simulink model "TwoButtonReaction"  (R2023b)
settings: Solver=FixedStepAuto  StartTime=0.0  StopTime=Inf  FixedStep=0.001  RelTol=1e-3  EnableMultiTasking=on
libraries: arduinolib x5
settings Model: ExtModeTrigDuration=2  Creator=vboutrou  LastModifiedBy=vboutrou
settings DataIOCC: DSMLogging=off  SaveTime=off  ReturnWorkspaceOutputs=off
settings OptimizationCC: EnhancedBackFolding=on  PassReuseOutputArgsAs=Individual arguments  ZeroExternalMemoryAtStartup=off  ZeroInternalMemoryAtStartup=off  MaxStackSize=64  OptimizeBlockOrder=speed  DifferentSizesBufferReuse=on  OptimizationCustomize=off  EfficientTunableParamExpr=on
settings DebuggingCC: ParameterTunabilityLossMsg=error
settings HardwareCC: ProdBitPerInt=16  ProdBitPerPointer=16  ProdBitPerSizeT=16  ProdBitPerPtrDiffT=16  ProdLargestAtomicFloat=None  ProdWordSize=8  ProdHWDeviceType=Atmel->AVR
settings SFSimCC: MATLABDynamicMemAlloc=off
settings RTWCC: Description=Embedded Coder  SystemTargetFile=ert.tlc  HardwareBoard=Arduino Uno  TemplateMakefile=ert_default_tmf  Toolchain=Arduino AVR  BuildConfiguration=Faster Runs
settings CodeAppCC: ForceParamTrailComments=on  IgnoreCustomStorageClasses=off  MaxIdLength=95  OperatorAnnotations=on  SimulinkDataObjDesc=on  SFDataObjDesc=on  InsertBlockDesc=on
settings ERTTargetCC: SupportContinuousTime=on  SupportVariableSizeSignals=on  ExtModeTransport=3  ExtModeStaticAlloc=on  ExtModeAutomaticAllocSize=off  ExtModeStaticAllocSize=250  ExtModeMexFile=ext_xcp  ExtModeIntrfLevel=Level2 - Open

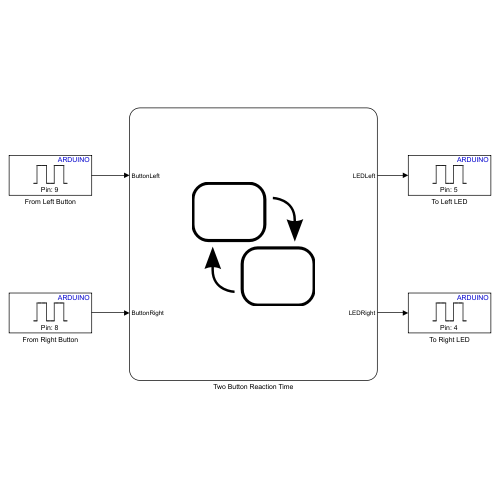
[thumbnail: Simulink's stored preview of the top-level diagram]
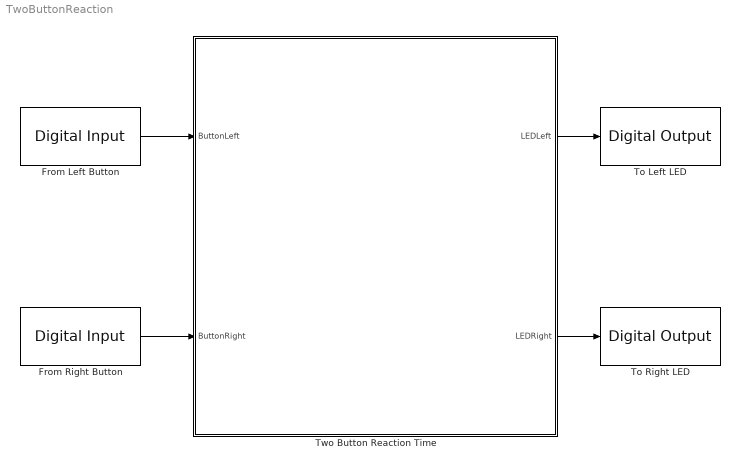
== system TwoButtonReaction ==
  From Left Button : arduinolib/Digital Input  pinNumber=9  mode=Default  Direction=input  SampleTime=-1  blockPlatform=arduino
  From Right Button : arduinolib/Digital Input  pinNumber=8  mode=Default  Direction=input  SampleTime=-1  blockPlatform=arduino
  To Left LED : arduinolib/Digital Output  pinNumber=5  Direction=output  blockPlatform=arduino
  To Right LED : arduinolib/Digital Output  pinNumber=4  Direction=output  blockPlatform=arduino
  Two Button Reaction Time : Stateflow chart  TreatAsAtomicUnit=on
  wires:
  From Left Button/1 -> Two Button Reaction Time/1(ButtonLeft)
  Two Button Reaction Time/1(LEDLeft) -> To Left LED/1
  From Right Button/1 -> Two Button Reaction Time/2(ButtonRight)
  Two Button Reaction Time/2(LEDRight) -> To Right LED/1

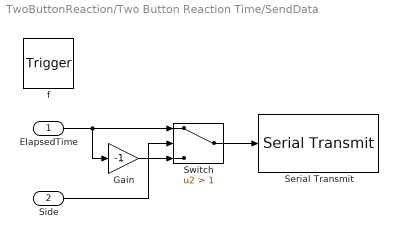
== system TwoButtonReaction/Two Button Reaction Time/SendData ==
  ElapsedTime : Inport  OutDataTypeStr=double  PortDimensions=1
  Side : Inport  Port=2  OutDataTypeStr=double  PortDimensions=1
  f : TriggerPort  TriggerType=function-call  VariantControl=(inherit)
      settings: CopyFcn=Stateflow.SLINSF.SimulinkMan.removeBlockPreDeleteFcn  PreDeleteFcn=Stateflow.SLINSF.SimulinkMan.unsafePredeleteFcn
  Gain : Gain  Gain=-1
  Serial Transmit : arduinolib/Serial Transmit  portNumber=0  sendmode=println  sendformat=Decimal  floatprecision=2  blockPlatform=arduino
  Switch : Switch  Criteria=u2 > Threshold  Threshold=1  SaturateOnIntegerOverflow=off  InputSameDT=off
  wires:
  Side/1 -> Switch/2
  ElapsedTime/1 -> Switch/1, Gain/1
  Gain/1 -> Switch/3
  Switch/1 -> Serial Transmit/1

== stateflow chart TwoButtonReaction/Two Button Reaction Time ==
  state SendData(ElapsedTime,Side) [function]
  state InitialState
    entry:
    Step = 0; % First step
    LEDRight = 1; % Right LED turned on
    LEDLeft = 1; % Left LED turned off
  state GameOn
    entry:
    LEDRight = 0;
    LEDLeft = 0;
    Step = Step + 1;
    Side = LeftRightSequence(Step);
    TimeStep = TimeStepSequence(Step);
  state TurnOnLeft
    en:
    LEDLeft = 1;
    LEDRight = 0;
    en,du:
    ElapsedTime = temporalCount(msec);
  state TurnOnRight
    en:
    LEDRight = 1;
    LEDLeft = 0;
    en,du:
    ElapsedTime = temporalCount(msec);
  state SendDataBack
    en:
    LEDLeft = 0;
    LEDRight = 0;
    SendData(ElapsedTime,Side)
  (default) -> InitialState
  InitialState -> GameOn : [ButtonRight & ButtonLeft]
  SendDataBack -> GameOn
  GameOn -> (junction 73) : after(TimeStep,sec)
  (junction 73) -> TurnOnLeft [order 2] : [Side == 1]
  (junction 73) -> TurnOnRight [order 1] : [Side==2]
  TurnOnLeft -> (junction 93) : [ButtonLeft==1]
  TurnOnRight -> (junction 93) : [ButtonRight==1]
  (junction 93) -> SendDataBack
  data: ElapsedTime function_input double size=1; Side function_input double size=1; u function_input; y function_output; u function_input; y function_output; ButtonLeft input; LEDLeft output; ButtonRight input; LEDRight output; ElapsedTime local; Side local; Step local; TimeStep local
  function y = LeftRightSequence(u):
    | function y = LeftRightSequence(u)
    |     Sequence = [1,1,2,2,2,1,2,1,1,2,2,2,2,1,2,1,2,1,1,1,1,2,1,1,2,2,1,2,1,1,2,2,2,1,1,1,1,1,2,2,1,1,2,2,2,...
    |         2,2,2,2,1,2,1,1,1,1,1,2,1,1,2,2,2,1,2,1,2,1,1,1,1,1,2,1,1,2,2,1,1,2,2,1,1,2,1,2,2,2,2,1,1,1,1,1,1,...
    |         1,2,2,2,2,2,1,1,2,1,1,2,2,2,1,1,1,1,1,1,1,1,1,2,1,2,1,1,1,2,2,2,1,2,1,1,1,2,1,2,1,1,2,1,2,1,1,1,1,...
    |         2,1,2,2,1,2,2,1,2,2,2,1,1,2,1,2,1,2,2,1,2,2,1,1,1,1,2,2,2,2,1,1,1,1,1,2,1,1,2,1,1,2,1,1,2,2,2,2,2,...
    |         1,1,2,2,2,2,1,1];
    |     id = mod(u,200);
    |     y = Sequence(id);
    | end
  function y = TimeStepSequence(u):
    | function y = TimeStepSequence(u)
    |     Sequence = [1.0387,1.4772,1.0461,1.4431,1.4291,0.8904,0.7672,1.0966,0.9758,1.2830,1.0576,0.8140,0.8051,...
    |         1.6737,0.8665,0.8686,1.5167,1.3664,1.0298,1.0700,1.5522,1.0704,1.2664,0.9011,1.6204,1.0825,1.1669,...
    |         1.0022,1.1312,0.9421,1.6224,1.6284,0.7975,0.9517,0.7650,0.7824,1.0708,1.2186,1.2764,1.0276,1.4089,...
    |         1.2953,1.0552,0.7489,1.1722,1.5272,1.1622,1.0490,1.4562,1.6274,0.8767,0.9374,0.9322,1.3733,1.5636,...
    |         1.4845,0.9302,1.6035,1.1068,0.7342,1.4143,1.0610,1.3334,0.8567,1.4376,1.4558,1.2664,1.4621,1.4517,...
    |         0.9682,1.0294,1.1071,1.6755,1.1364,1.6454,1.2611,1.1402,0.8946,1.6959,1.3670,1.6311,1.6407,1.5759,...
    |         1.2712,1.4302,1.2246,0.8356,1.1758,1.1918,1.3367,1.4680,1.5298,0.9371,1.3299,1.1787,0.9942,1.0264,...
    |         1.6746,0.7520,0.9331,1.5772,1.6181,1.0224,0.8805,0.8953,0.8407,1.4422,1.5359,0.9922,1.0829,1.6107,...
    |         1.1434,1.0196,1.4425,0.8665,1.3764,1.6986,1.1025,0.8641,1.0868,0.7532,1.4251,1.2224,1.2922,1.6245,...
    |         1.2085,1.0011,1.0975,0.9791,1.4864,1.5835,1.3350,1.1288,1.2458,0.7748,1.4122,0.8190,0.8767,0.7280,...
    |         1.3206,1.1038,1.6197,1.1927,0.9702,1.4091,1.2877,1.1015,0.7123,0.9691,1.3518,1.3457,1.6695,0.7484,...
    |         1.2143,1.4490,1.5548,1.6221,1.6572,1.0987,1.4336,0.7410,1.0681,1.1590,1.5178,1.3520,1.0039,1.1346,...
    |         1.0603,1.4663,1.4273,1.1037,1.4900,1.3790,1.5435,0.7665,1.4628,1.1941,1.4211,1.1947,1.2906,1.6607,...
    |         0.7148,1.6352,0.9582,1.0579,0.7186,1.6606,1.4514,1.4360,1.6543,0.7474,1.1017,1.3861,1.2913,1.3708,...
    |         1.1968,1.4424,1.6191,1.6543,0.7472];
    |     id = mod(u,200);
    |     y = Sequence(id);
    | end
